simulink library "pm_machines_library"  (Simulink 8.1)
settings: Solver=ode45  StartTime=0.0  StopTime=10.0  RelTol=1e-3
libraries: powerlib x6, powerlib_extras x3, pm_machines_library x2
settings Model: Creator=s0237326  LastModifiedBy=s0237326

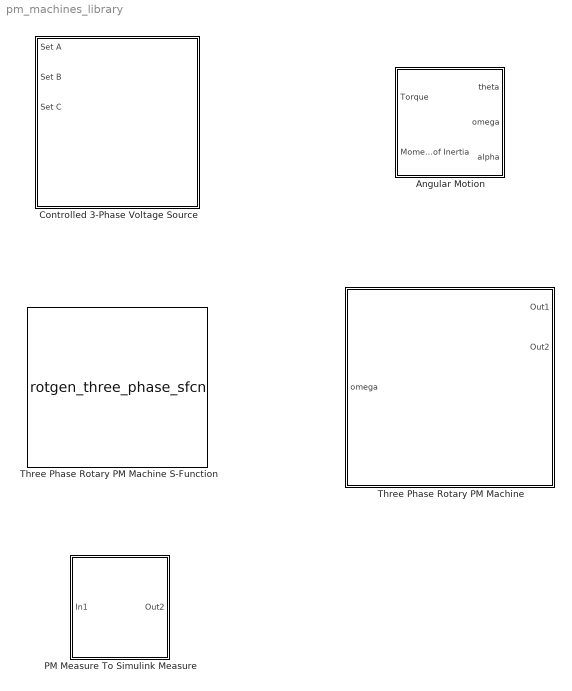
== system pm_machines_library ==
  Angular Motion : Subsystem
  Controlled 3-Phase Voltage Source : Subsystem  mask(Controlled 3-Phase Voltage Source){}
      mask help: Controlled 3-Phase Voltage Source Mask
  PM Measure To Simulink Measure : Subsystem  mask{ref_type=Stationary}
      mask prompts: ref_type "dq Reference Type"
      mask TypeOptions ref_type: Synchronous | Stationary
  Three Phase Rotary PM Machine : Subsystem
      mask Display:
      | port_label('input', 1, 'Omega')
      | port_label('output', 1, 'Torque')
      | port_label('output', 2, 'Meas')
      | port_label('rconn', 1, 'Phase A')
      | port_label('rconn', 2, 'Phase B')
      | port_label('rconn', 3, 'Phase C')
  Three Phase Rotary PM Machine S-Function : M-S-Function  FunctionName=rotgen_three_phase_sfcn
      mask Display:
      | port_label('input', 1, 'theta')
      | port_label('input', 2, 'omega')
      | port_label('input', 3, 'Phase A Current')
      | port_label('input', 4, 'Phase B Current')
      | port_label('input', 5, 'Phase C Current')
      | port_label('output', 1, 'Torque')
      | port_label('output', 2, 'Phase A EMF')
      | port_label('output', 3, 'Phase B EMF')
      | port_label('output', 4, 'Phase C EMF')
      | port_label('output', 5, 'Meas')

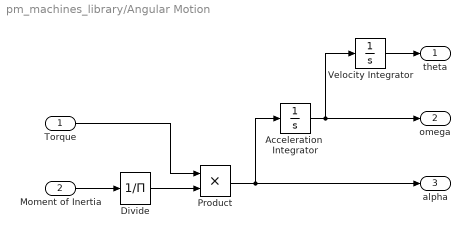
== system pm_machines_library/Angular Motion ==
  Torque : Inport
  Moment of Inertia : Inport  Port=2
  Acceleration  Integrator : Integrator
  Divide : Product  Inputs=/
  Product : Product  RndMeth=Zero
  Velocity Integrator : Integrator
  theta : Outport
  omega : Outport  Port=2
  alpha : Outport  Port=3
  wires:
  Product/1 -> alpha/1, Acceleration  Integrator/1
  Velocity Integrator/1 -> theta/1
  Acceleration  Integrator/1 -> omega/1, Velocity Integrator/1
  Torque/1 -> Product/1
  Moment of Inertia/1 -> Divide/1
  Divide/1 -> Product/2

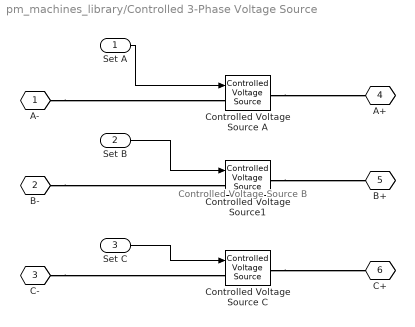
== system pm_machines_library/Controlled 3-Phase Voltage Source ==
  note: Controlled Voltage Source B
  Set A : Inport  PortDimensions=1
  Set B : Inport  Port=2  PortDimensions=1
  Set C : Inport  Port=3  PortDimensions=1
  Controlled Voltage Source A : powerlib/Electrical Sources/Controlled Voltage Source  Initialize=off  Source_Type=AC  Amplitude=0  Phase=0  Frequency=0  Measurements=None
  Controlled Voltage Source C : powerlib/Electrical Sources/Controlled Voltage Source  Initialize=off  Source_Type=AC  Amplitude=0  Phase=0  Frequency=0  Measurements=None
  Controlled Voltage Source1 : powerlib/Electrical Sources/Controlled Voltage Source  Initialize=off  Source_Type=AC  Amplitude=0  Phase=0  Frequency=0  Measurements=None
  A- : PMIOPort  Tag=PMCPort  Port=1  Side=Left
  B- : PMIOPort  Tag=PMCPort  Port=2  Side=Left
  C- : PMIOPort  Tag=PMCPort  Port=3  Side=Left
  A+ : PMIOPort  Tag=PMCPort  Port=4  Side=Right
  B+ : PMIOPort  Tag=PMCPort  Port=5  Side=Right
  C+ : PMIOPort  Tag=PMCPort  Port=6  Side=Right
  wires:
  Set C/1 -> Controlled Voltage Source C/1
  Set B/1 -> Controlled Voltage Source1/1
  Set A/1 -> Controlled Voltage Source A/1
  connections:
  A-/RConn1 -- Controlled Voltage Source A/LConn1
  Controlled Voltage Source A/RConn1 -- A+/RConn1
  C-/RConn1 -- Controlled Voltage Source C/LConn1
  Controlled Voltage Source C/RConn1 -- C+/RConn1
  B-/RConn1 -- Controlled Voltage Source1/LConn1
  Controlled Voltage Source1/RConn1 -- B+/RConn1

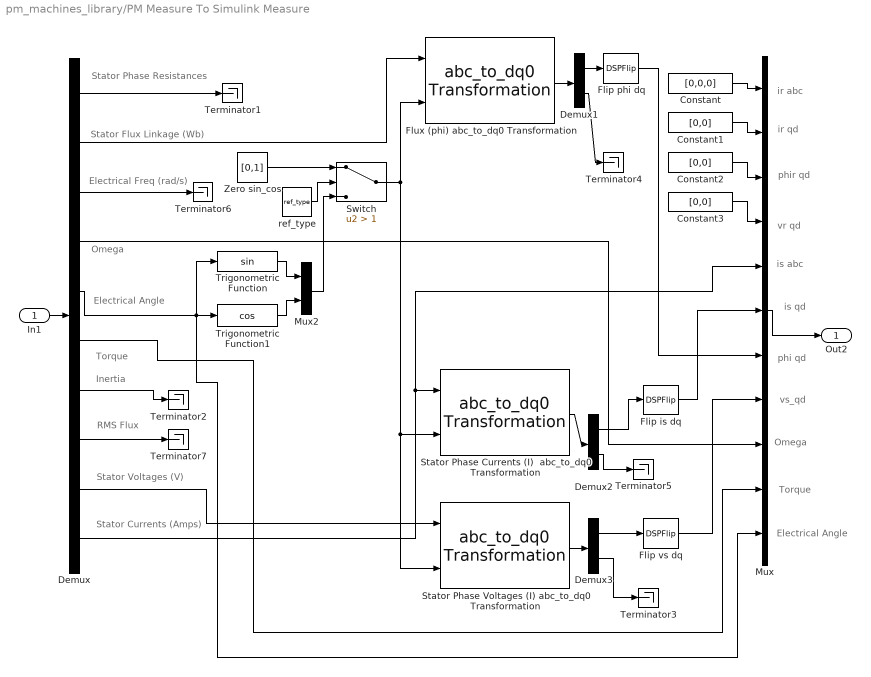
== system pm_machines_library/PM Measure To Simulink Measure ==
  note: RMS Flux
  note: Electrical Freq (rad/s)
  note: Stator Flux Linkage (Wb)
  note: Stator Currents (Amps)
  note: Stator Voltages (V)
  note: Omega
  note: Electrical Angle
  note: Torque
  note: Torque
  note: Omega
  note: vs_qd
  note: is qd
  note: phi qd
  note: is abc
  note: ir abc
  note: ir qd
  note: phir qd
  note: vr qd
  note: Stator Phase Resistances
  note: Inertia
  note: Electrical Angle
  In1 : Inport
  Constant : Constant  Value=[0,0,0]
  Constant1 : Constant  Value=[0,0]
  Constant2 : Constant  Value=[0,0]
  Constant3 : Constant  Value=[0,0]
  Demux : Demux  Outputs=[3, 3, 1, 1, 1, 1, 1, 1, 3, 3]
  Demux1 : Demux  Outputs=[2,1]
  Demux2 : Demux  Outputs=[2,1]
  Demux3 : Demux  Outputs=[2,1]
  Flip is dq : DSPFlip
  Flip phi dq : DSPFlip
  Flip vs dq : DSPFlip
  Flux (phi) abc_to_dq0 Transformation : powerlib_extras/Measurements/abc_to_dq0 Transformation
  Mux : Mux  Inputs=11
  Mux2 : Mux  Inputs=2
  Stator Phase Currents (I)  abc_to_dq0 Transformation : powerlib_extras/Measurements/abc_to_dq0 Transformation
  Stator Phase Voltages (I) abc_to_dq0 Transformation : powerlib_extras/Measurements/abc_to_dq0 Transformation
  Switch : Switch  Criteria=u2 > Threshold  Threshold=1  ZeroCross=off
  Terminator{1..7} (7 alike) : Terminator
  Trigonometric Function : Trigonometry
  Trigonometric Function1 : Trigonometry  Operator=cos
  Zero sin_cos : Constant  Value=[0,1]
  ref_type : Constant  Value=ref_type
  Out2 : Outport
  wires:
  Demux/2 -> Flux (phi) abc_to_dq0 Transformation/1
  In1/1 -> Demux/1
  Demux/4 -> Mux/9
  Demux/6 -> Mux/10
  Mux/1 -> Out2/1
  Demux/1 -> Terminator1/1
  Demux/9 -> Stator Phase Voltages (I) abc_to_dq0 Transformation/1
  Demux/10 -> Stator Phase Currents (I)  abc_to_dq0 Transformation/1, Mux/5
  Demux/7 -> Terminator2/1
  Demux/5 -> Mux/11, Trigonometric Function/1, Trigonometric Function1/1
  Trigonometric Function/1 -> Mux2/1
  Trigonometric Function1/1 -> Mux2/2
  Flux (phi) abc_to_dq0 Transformation/1 -> Demux1/1
  Stator Phase Currents (I)  abc_to_dq0 Transformation/1 -> Demux2/1
  Stator Phase Voltages (I) abc_to_dq0 Transformation/1 -> Demux3/1
  Constant/1 -> Mux/1
  Constant3/1 -> Mux/4
  Constant2/1 -> Mux/3
  Constant1/1 -> Mux/2
  Flip is dq/1 -> Mux/6
  Demux2/1 -> Flip is dq/1
  Demux3/1 -> Flip vs dq/1
  Flip vs dq/1 -> Mux/8
  Demux1/1 -> Flip phi dq/1
  Flip phi dq/1 -> Mux/7
  Demux3/2 -> Terminator3/1
  Demux1/2 -> Terminator4/1
  Demux2/2 -> Terminator5/1
  Demux/3 -> Terminator6/1
  Zero sin_cos/1 -> Switch/1
  Mux2/1 -> Switch/3
  ref_type/1 -> Switch/2
  Switch/1 -> Stator Phase Currents (I)  abc_to_dq0 Transformation/2, Stator Phase Voltages (I) abc_to_dq0 Transformation/2, Flux (phi) abc_to_dq0 Transformation/2
  Demux/8 -> Terminator7/1

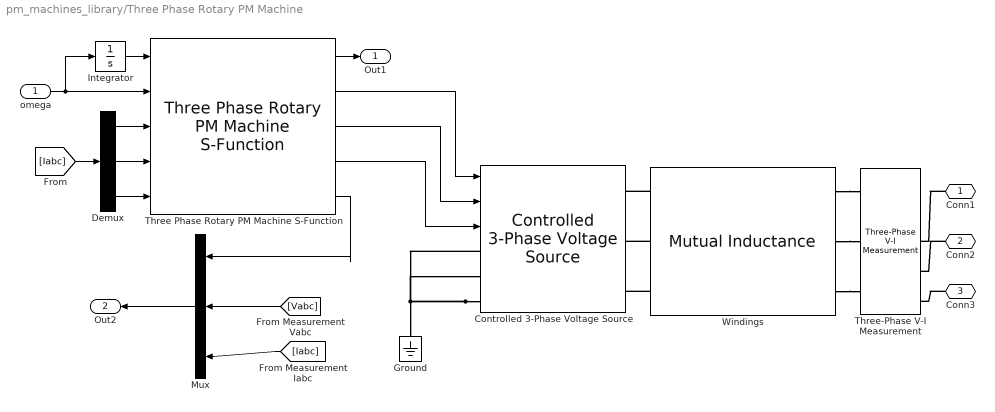
== system pm_machines_library/Three Phase Rotary PM Machine ==
  omega : Inport
  Controlled 3-Phase Voltage Source : pm_machines_library/Controlled 3-Phase Voltage Source
  Demux : Demux  Outputs=3
  Ground : powerlib/Elements/Ground  LConnTagsString=a
  Integrator : Integrator
  Mux : Mux  Inputs=3
  Three Phase Rotary PM Machine S-Function : pm_machines_library/Three Phase Rotary PM Machine S-Function
  Three-Phase V-I Measurement : powerlib/Measurements/Three-Phase V-I Measurement  VoltageMeasurement=phase-to-ground  SetLabelV=on  LabelV=Vabc  Vpu=off  VpuLL=off  CurrentMeasurement=yes  SetLabelI=on  LabelI=Iabc  Ipu=off  Pbase=100e6  Vbase=500e3  OutputType=Complex  PhasorSimulation=off  PSBequivalent=0
  Windings : powerlib/Elements/Mutual Inductance  LConnTagsString=a|b|c  RConnTagsString=A|B|C  TypeOfMutual=Two or three windings with equal mutual terms  NumberOfWindings=3  SelfImpedance1=[1.1 1.1e-03]  SelfImpedance2=[ 1.1 1.1e-03]  ThreeWindings=on  SelfImpedance3=[ 1.1 1.1e-03]  MutualImpedance=[1.0 1.0e-03]  InductanceMatrix="[1.0 0.9  0.9 ;  0.9 1.0  0.9;  0.9 0.9 1.0 ] * 1e-3"  ResistanceMatrix="[1.0 0.9  0.9 ;  0.9 1.0  0.9;  0.9 0.9 1.0 ]"  Measurements=None
      settings: AttributesFormatString=\n
  Conn1 : PMIOPort  Port=1  Side=Right
  Conn2 : PMIOPort  Port=2  Side=Right
  Conn3 : PMIOPort  Port=3  Side=Right
  Out1 : Outport
  Out2 : Outport  Port=2
  wires:
  Demux/3 -> Three Phase Rotary PM Machine S-Function/5
  Demux/2 -> Three Phase Rotary PM Machine S-Function/4
  Demux/1 -> Three Phase Rotary PM Machine S-Function/3
  [Iabc] -> Demux/1
  Three Phase Rotary PM Machine S-Function/4 -> Controlled 3-Phase Voltage Source/3
  Three Phase Rotary PM Machine S-Function/3 -> Controlled 3-Phase Voltage Source/2
  Three Phase Rotary PM Machine S-Function/2 -> Controlled 3-Phase Voltage Source/1
  Integrator/1 -> Three Phase Rotary PM Machine S-Function/1
  omega/1 -> Three Phase Rotary PM Machine S-Function/2, Integrator/1
  Three Phase Rotary PM Machine S-Function/1 -> Out1/1
  Three Phase Rotary PM Machine S-Function/5 -> Mux/1
  [Vabc] -> Mux/2
  [Iabc] -> Mux/3
  Mux/1 -> Out2/1
  connections:
  Controlled 3-Phase Voltage Source/LConn3 -- Controlled 3-Phase Voltage Source/LConn2 -- Controlled 3-Phase Voltage Source/LConn1 -- Ground/LConn1
  Windings/LConn1 -- Controlled 3-Phase Voltage Source/RConn1
  Windings/LConn2 -- Controlled 3-Phase Voltage Source/RConn2
  Windings/LConn3 -- Controlled 3-Phase Voltage Source/RConn3
  Windings/RConn1 -- Three-Phase V-I Measurement/LConn1
  Windings/RConn2 -- Three-Phase V-I Measurement/LConn2
  Windings/RConn3 -- Three-Phase V-I Measurement/LConn3
  Conn1/RConn1 -- Three-Phase V-I Measurement/RConn1
  Conn2/RConn1 -- Three-Phase V-I Measurement/RConn2
  Conn3/RConn1 -- Three-Phase V-I Measurement/RConn3
